simulink model "manual_waveInput"  (R2023a)
settings: Solver=FixedStepAuto  StartTime=0.0  StopTime=inf  FixedStep=0.01  RelTol=1e-3  EnableMultiTasking=on
undefined symbols (not defined in the file): dev, Main, mf, P0, pwm_output0, Q, R, Rbody_frd, Ts_EKF_integr, Ts_EKF_meas, Ts_slk, x0EKF
libraries: simulink_extras x6, px4Sensorslib x4, sharedtransform x4, px4lib x1, px4uORBlib x1
settings Model: SimulationMode=external  ExtModeTrigDuration=10  Creator=ArriGE66  LastModifiedBy=User
settings SolverCC: PositivePriorityOrder=on
settings OptimizationCC: EnhancedBackFolding=on  PassReuseOutputArgsAs=Individual arguments  ZeroExternalMemoryAtStartup=off  ZeroInternalMemoryAtStartup=off  MaxStackSize=64  OptimizeBlockOrder=speed  DifferentSizesBufferReuse=on  OptimizationCustomize=off  EfficientTunableParamExpr=on
settings DebuggingCC: ParameterTunabilityLossMsg=error
settings HardwareCC: ProdBitPerPointer=32  ProdBitPerSizeT=32  ProdBitPerPtrDiffT=32  ProdLargestAtomicInteger=Long  ProdLargestAtomicFloat=Double  ProdWordSize=32  ProdLongLongMode=on  ProdHWDeviceType=ARM Compatible->ARM Cortex
settings SFSimCC: MATLABDynamicMemAlloc=off  SimTargetLang=C++
settings RTWCC: Description=Embedded Coder  SystemTargetFile=ert.tlc  HardwareBoard=PX4 Cube Orange  TemplateMakefile=ert_default_tmf  Toolchain=GNU Tools for PX4 Autopilots  TargetLang=C++
settings CodeAppCC: ForceParamTrailComments=on  IgnoreCustomStorageClasses=off  OperatorAnnotations=on  SimulinkDataObjDesc=on  SFDataObjDesc=on  InsertBlockDesc=on
settings ERTTargetCC: ExtMode=on  ExtModeTransport=3  ExtModeStaticAlloc=on  ExtModeStaticAllocSize=1024  ExtModeMexFile=ext_xcp  ExtModeMexArgs=1 COM10 3000000  ExtModeIntrfLevel=Level2 - Open

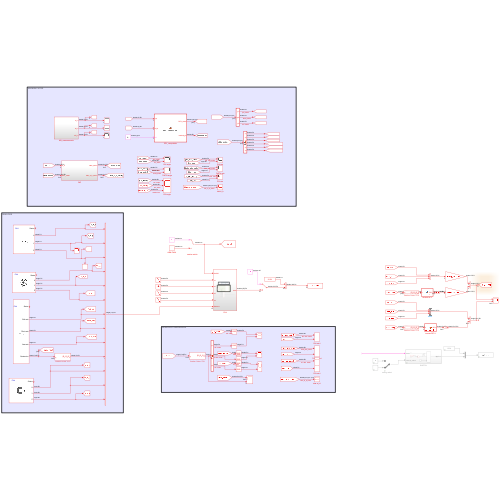
[thumbnail: Simulink's stored preview of the top-level diagram]
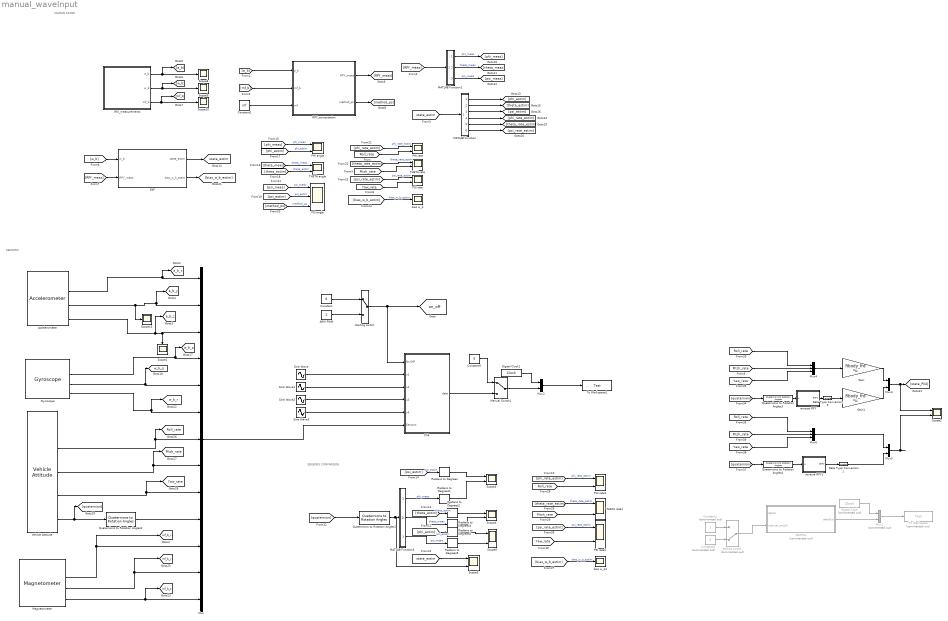
== system manual_waveInput ==
  note: KALMAN FILTER
  note: SENSORS
  note: SENSORS COMPARISON
  ARM PWM : Constant  OutDataTypeStr=boolean  SampleTime=0.01
  Accelerometer : px4Sensorslib/Accelerometer  uorbTimeStamp=off  BlockingMode=off  BlockTimeout=1e-3  sampleTime=1/100
  Constant : Constant  Value=0  OutDataTypeStr=boolean
  Constant1 : Constant  Commented=on  OutDataTypeStr=boolean
  Constant2 : Constant  Value=mf
  Constant3 : Constant  Commented=on  Value=0  OutDataTypeStr=boolean
  Constant5 : Constant  Value=0  OutDataTypeStr=boolean
  Data Type Conversion1 : DataTypeConversion  OutDataTypeStr=single  SaturateOnIntegerOverflow=off  RndMeth=Floor
  Data Type Conversion5 : DataTypeConversion  OutDataTypeStr=single  SaturateOnIntegerOverflow=off  RndMeth=Floor
  Digital Clock : DigitalClock  Commented=on  SampleTime=0.01
  Digital Clock1 : DigitalClock  SampleTime=0.01
  EKF : Subsystem
  Gain : Gain  Gain=Rbody_frd  Multiplication=Matrix(K*u) (u vector)
  Gain1 : Gain  Gain=Rbody_frd  Multiplication=Matrix(K*u) (u vector)
  Gyroscope : px4Sensorslib/Gyroscope  uorbTimeStamp=off  BlockingMode=off  BlockTimeout=1e-3  sampleTime=1/100
  IMU_measurements : Subsystem
  MATLAB Function : MATLAB Function  TreatAsAtomicUnit=on
  MATLAB Function1 : MATLAB Function  TreatAsAtomicUnit=on
  MATLAB Function3 : MATLAB Function  TreatAsAtomicUnit=on
  Magnetometer : px4Sensorslib/Magnetometer  uorbTimeStamp=off  BlockingMode=off  BlockTimeout=1e-3  sampleTime=0.01
  Manual Switch1 : ManualSwitch
  Mux : Mux  Inputs=13
  Mux1 : Mux  Commented=on  Inputs=2
  Mux2 : Mux  Inputs=2
  Mux3 : Mux  Inputs=2
  Mux4 : Mux  Inputs=3
  Mux5 : Mux  Inputs=2
  Mux6 : Mux  Inputs=3
  PHI angle : Scope  NumInputPorts=2
  PHI rate : Scope  NumInputPorts=2
  PHI rate1 : Scope  NumInputPorts=2
  PSI angle : Scope  NumInputPorts=3
  PSI rate : Scope  NumInputPorts=2
  PSI rate1 : Scope  NumInputPorts=2
  PX4 : Subsystem
  Quaternions to Rotation Angles{1..4} (4 alike) : sharedtransform/Quaternions to Rotation Angles  rotationOrder=ZYX  aMode=aMode
  RPY_computation : MATLAB Function  TreatAsAtomicUnit=on
  Radians to Degrees{,1..5} (6 alike) : simulink_extras/Transformations/Radians to Degrees
  SWITCH : Subsystem  Commented=on
  Scope{1,8..10,13} (5 alike) : Scope
  Scope{2..6} (5 alike) : Scope  NumInputPorts=2
  Sine Wave : Sin  Amplitude=0  SampleTime=0.01
  Sine Wave1 : Sin  Amplitude=0  Phase=pi/2  SampleTime=0.01
  Sine Wave2 : Sin  Amplitude=200  Bias=300  SampleTime=0.01
  Sine Wave3 : Sin  Amplitude=200  Bias=300  Phase=pi/2  SampleTime=0.01
  THETA angle : Scope  NumInputPorts=2
  THETA rate : Scope  NumInputPorts=2
  THETA rate1 : Scope  NumInputPorts=2
  To Workspace : ToWorkspace  Commented=on  VariableName=Test  SampleTime=0.01
      settings: Save2DSignal=2-D array (concatenate along first dimension)
  To Workspace1 : ToWorkspace  VariableName=Test  SampleTime=-1
      settings: Save2DSignal=2-D array (concatenate along first dimension)
  Vehicle Attitude : px4Sensorslib/Vehicle Attitude  rollRate=on  pitchRate=on  yawRate=on  quaternion=on  uorbTimeStamp=off  BlockingMode=off  BlockTimeout=0.001  sampleTime=1/100
  bias w_b : Scope
  bias w_b1 : Scope
  ending switch : ManualSwitch  Commented=on  CurrentSetting=0
  reverse RPY : MATLAB Function  TreatAsAtomicUnit=on
  reverse RPY1 : MATLAB Function  TreatAsAtomicUnit=on
  starting switch : ManualSwitch
  tag scope: Pitch_rate=global, Roll_rate=global, Yaw_rate=global, a_b_x=global, a_b_y=global, a_b_z=global, mf_b_x=global, mf_b_y=global, mf_b_z=global, on_off=global, state_estim=global, w_b_p=global, w_b_q=global, w_b_r=global
  wires:
  Vehicle Attitude/3 -> [Pitch_rate], Mux/8
  Vehicle Attitude/2 -> [Roll_rate], Mux/7
  ARM PWM/1 -> starting switch/2
  Constant/1 -> starting switch/1
  Gyroscope/4 -> [w_b_r], Mux/6
  Gyroscope/3 -> [w_b_q], Mux/5
  Gyroscope/2 -> [w_b_p], Mux/4
  Accelerometer/2 -> [a_b_x], Mux/1
  Accelerometer/3 -> Scope13/1, [a_b_y], Mux/2
  Accelerometer/4 -> [a_b_z], Mux/3, Scope1/1
  Vehicle Attitude/4 -> [Yaw_rate], Mux/9
  Magnetometer/2 -> [mf_b_x], Mux/11
  Magnetometer/3 -> Mux/12, [mf_b_y]
  Magnetometer/4 -> [mf_b_z], Mux/13
  MATLAB Function1/2(y2) -> [theta_meas]  "theta_meas"
  [bias_w_b_estim] -> bias w_b/1  "bias_w_b_estim"
  [mf_b] -> RPY_computation/2(mf_b)
  [theta_estim] -> THETA angle/2  "theta_estim"
  MATLAB Function1/1(y1) -> [phi_meas]  "phi_meas"
  [RPY_meas] -> EKF/2(RPY_meas)
  [psi_meas] -> PSI angle/1  "psi_meas"
  [method_ps] -> PSI angle/3  "method_ps"
  IMU_measurements/2(w_b) -> Scope9/1, [w_b]
  [psi_estim] -> PSI angle/2  "psi_estim"
  MATLAB Function1/3(y3) -> [psi_meas]  "psi_meas"
  [RPY_meas] -> MATLAB Function1/1(u)
  [theta_meas] -> THETA angle/1  "theta_meas"
  [phi_rate_estim] -> PHI rate/1  "phi_rate_estim"
  [psi_rate_estim] -> PSI rate/1  "psi_rate_estim"
  [theta_rate_estim] -> THETA rate/1  "theta_rate_estim"
  EKF/1(state_estim) -> [state_estim]
  [phi_estim] -> PHI angle/2  "phi_estim"
  [w_b] -> EKF/1(w_b)
  IMU_measurements/3(mf_b) -> [mf_b], Scope10/1
  Constant2/1 -> RPY_computation/3(mf)
  IMU_measurements/1(a_b) -> [a_b], Scope8/1
  RPY_computation/2(method_ps) -> [method_ps]
  [a_b] -> RPY_computation/1(a_b)
  EKF/2(bias_w_b_estim) -> [bias_w_b_estim]
  [phi_meas] -> PHI angle/1  "phi_meas"
  RPY_computation/1(RPY_meas) -> [RPY_meas]
  starting switch/1 -> PX4/1(On/Off), [on_off]
  Mux/1 -> PX4/6(Sensors)
  [state_estim] -> MATLAB Function/1(u)
  MATLAB Function/1(y1) -> [phi_estim]
  MATLAB Function/2(y2) -> [theta_estim]
  MATLAB Function/3(y3) -> [psi_estim]
  MATLAB Function/4(y4) -> [phi_rate_estim]
  MATLAB Function/5(y5) -> [theta_rate_estim]
  MATLAB Function/6(y6) -> [psi_rate_estim]
  Sine Wave/1 -> PX4/2(u1)
  Sine Wave1/1 -> PX4/3(u2)
  Sine Wave2/1 -> PX4/4(u3)
  Sine Wave3/1 -> PX4/5(u4)
  [Roll_rate] -> PHI rate/2
  [Pitch_rate] -> THETA rate/2
  [Yaw_rate] -> PSI rate/2
  [bias_w_b_estim] -> bias w_b1/1  "bias_w_b_estim"
  [psi_rate_estim] -> PSI rate1/1  "psi_rate_estim"
  Radians to Degrees2/1 -> Scope4/1
  [state_estim] -> Scope6/1
  [phi_estim] -> Radians to Degrees4/1  "phi_estim"
  MATLAB Function3/3(y3) -> Radians to Degrees5/1  "psi_meas"
  MATLAB Function3/1(y1) -> Radians to Degrees1/1  "phi_meas"
  [theta_estim] -> Radians to Degrees2/1  "theta_estim"
  Radians to Degrees1/1 -> Scope3/2
  Quaternions to Rotation Angles1/1 -> Scope6/2, MATLAB Function3/1(u)
  Radians to Degrees3/1 -> Scope4/2
  Radians to Degrees5/1 -> Scope5/2
  MATLAB Function3/2(y2) -> Radians to Degrees3/1  "theta_meas"
  Radians to Degrees/1 -> Scope3/1
  Radians to Degrees4/1 -> Scope5/1
  [Roll_rate] -> PHI rate1/2
  [psi_estim] -> Radians to Degrees/1  "psi_estim"
  [Yaw_rate] -> PSI rate1/2
  [theta_rate_estim] -> THETA rate1/1  "theta_rate_estim"
  [quaternion] -> Quaternions to Rotation Angles1/1
  [Pitch_rate] -> THETA rate1/2
  [phi_rate_estim] -> PHI rate1/1  "phi_rate_estim"
  Vehicle Attitude/5 -> [quaternion], Quaternions to Rotation Angles2/1
  Quaternions to Rotation Angles2/1 -> Mux/10
  Constant3/1 -> ending switch/2
  ? -> SWITCH/1(dataIn)
  ending switch/1 -> SWITCH/2(manual_switch)
  Constant1/1 -> ending switch/1
  Mux1/1 -> To Workspace/1
  Digital Clock/1 -> Mux1/1
  SWITCH/1(dataOut) -> Mux1/2
  Mux2/1 -> To Workspace1/1
  Constant5/1 -> Manual Switch1/1
  Digital Clock1/1 -> Mux2/1
  Manual Switch1/1 -> Mux2/2
  PX4/1(data) -> Manual Switch1/2
  [Pitch_rate] -> Mux4/2
  [Yaw_rate] -> Mux4/3
  Mux3/1 -> Scope2/1, [state_PX4]
  Data Type Conversion5/1 -> Gain1/1
  [Roll_rate] -> Mux4/1
  Quaternions to Rotation Angles3/1 -> reverse RPY/1(u)
  reverse RPY/1(RPY) -> Data Type Conversion5/1
  Gain/1 -> Mux3/1
  [quaternion] -> Quaternions to Rotation Angles3/1
  Mux4/1 -> Gain/1
  Gain1/1 -> Mux3/2
  Data Type Conversion1/1 -> Mux5/2
  Mux6/1 -> Mux5/1
  reverse RPY1/1(RPY) -> Data Type Conversion1/1
  Quaternions to Rotation Angles4/1 -> reverse RPY1/1(u)
  [quaternion] -> Quaternions to Rotation Angles4/1
  [Roll_rate] -> Mux6/1
  Mux5/1 -> Scope2/2
  [Pitch_rate] -> Mux6/2
  [Yaw_rate] -> Mux6/3

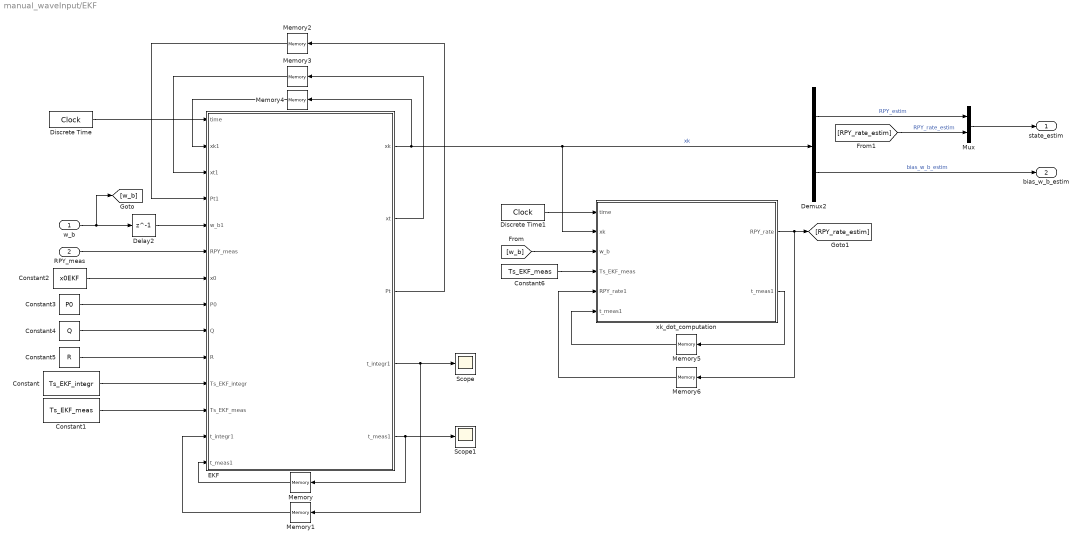
== system manual_waveInput/EKF ==
  w_b : Inport
  RPY_meas : Inport  Port=2
  Constant : Constant  Value=Ts_EKF_integr
  Constant1 : Constant  Value=Ts_EKF_meas
  Constant2 : Constant  Value=x0EKF
  Constant3 : Constant  Value=P0
  Constant4 : Constant  Value=Q
  Constant5 : Constant  Value=R
  Constant6 : Constant  Value=Ts_EKF_meas
  Delay2 : Delay  DelayLength=1  SampleTime=Ts_EKF_integr
  Demux2 : Demux  Outputs=2
  Discrete Time : DigitalClock  SampleTime=Ts_slk
  Discrete Time1 : DigitalClock  SampleTime=Ts_slk
  EKF : MATLAB Function  TreatAsAtomicUnit=on
  Memory{,1..6} (7 alike) : Memory
  Mux : Mux  Inputs=2
  Scope : Scope
  Scope1 : Scope
  xk_dot_computation : MATLAB Function  TreatAsAtomicUnit=on
  state_estim : Outport
  bias_w_b_estim : Outport  Port=2
  wires:
  w_b/1 -> Delay2/1, [w_b]
  Constant4/1 -> EKF/9(Q)
  Constant2/1 -> EKF/7(x0)
  Constant5/1 -> EKF/10(R)
  Memory/1 -> EKF/14("t_meas1 ")
  EKF/2(xt) -> Memory3/1
  Memory2/1 -> EKF/4(Pt1)
  EKF/3(Pt) -> Memory2/1
  RPY_meas/1 -> EKF/6(RPY_meas)
  Discrete Time/1 -> EKF/1(time)
  Memory3/1 -> EKF/3(xt1)
  Memory1/1 -> EKF/13("t_integr1 ")
  Constant3/1 -> EKF/8(P0)
  EKF/5(t_meas1) -> Scope1/1, Memory/1
  EKF/4(t_integr1) -> Scope/1, Memory1/1
  Delay2/1 -> EKF/5(w_b1)
  Constant/1 -> EKF/11(Ts_EKF_integr)
  Constant1/1 -> EKF/12(Ts_EKF_meas)
  Memory4/1 -> EKF/2(xk1)
  xk_dot_computation/2(t_meas1) -> Memory5/1
  Memory5/1 -> xk_dot_computation/6("t_meas1 ")
  Memory6/1 -> xk_dot_computation/5(RPY_rate1)
  xk_dot_computation/1(RPY_rate) -> [RPY_rate_estim], Memory6/1
  [w_b] -> xk_dot_computation/3(w_b)
  Discrete Time1/1 -> xk_dot_computation/1(time)
  Demux2/2 -> bias_w_b_estim/1  "bias_w_b_estim"
  Demux2/1 -> Mux/1  "RPY_estim"
  EKF/1(xk) -> xk_dot_computation/2(xk), Demux2/1, Memory4/1  "xk"
  [RPY_rate_estim] -> Mux/2  "RPY_rate_estim"
  Constant6/1 -> xk_dot_computation/4(Ts_EKF_meas)
  Mux/1 -> state_estim/1

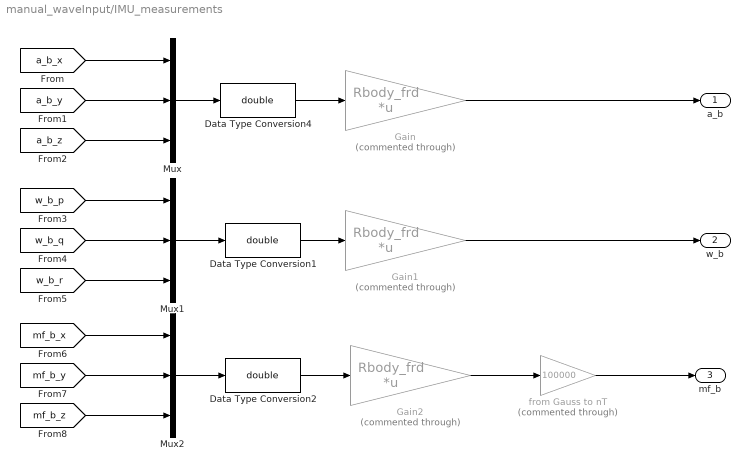
== system manual_waveInput/IMU_measurements ==
  Data Type Conversion1 : DataTypeConversion  OutDataTypeStr=double  SaturateOnIntegerOverflow=off  RndMeth=Floor
  Data Type Conversion2 : DataTypeConversion  OutDataTypeStr=double  SaturateOnIntegerOverflow=off  RndMeth=Floor
  Data Type Conversion4 : DataTypeConversion  OutDataTypeStr=double  SaturateOnIntegerOverflow=off  RndMeth=Floor
  Gain : Gain  Commented=through  Gain=Rbody_frd  Multiplication=Matrix(K*u) (u vector)
  Gain1 : Gain  Commented=through  Gain=Rbody_frd  Multiplication=Matrix(K*u) (u vector)
  Gain2 : Gain  Commented=through  Gain=Rbody_frd  Multiplication=Matrix(K*u) (u vector)
  Mux : Mux  Inputs=3
  Mux1 : Mux  Inputs=3
  Mux2 : Mux  Inputs=3
  from Gauss to nT : Gain  Commented=through  Gain=100000
  a_b : Outport
  w_b : Outport  Port=2
  mf_b : Outport  Port=3
  wires:
  Gain2/1 -> from Gauss to nT/1
  Mux2/1 -> Data Type Conversion2/1
  [a_b_x] -> Mux/1
  [a_b_y] -> Mux/2
  [a_b_z] -> Mux/3
  Mux/1 -> Data Type Conversion4/1
  Mux1/1 -> Data Type Conversion1/1
  [w_b_p] -> Mux1/1
  [w_b_r] -> Mux1/3
  [w_b_q] -> Mux1/2
  [mf_b_x] -> Mux2/1
  [mf_b_z] -> Mux2/3
  [mf_b_y] -> Mux2/2
  Gain/1 -> a_b/1
  Gain1/1 -> w_b/1
  from Gauss to nT/1 -> mf_b/1
  Data Type Conversion4/1 -> Gain/1
  Data Type Conversion1/1 -> Gain1/1
  Data Type Conversion2/1 -> Gain2/1

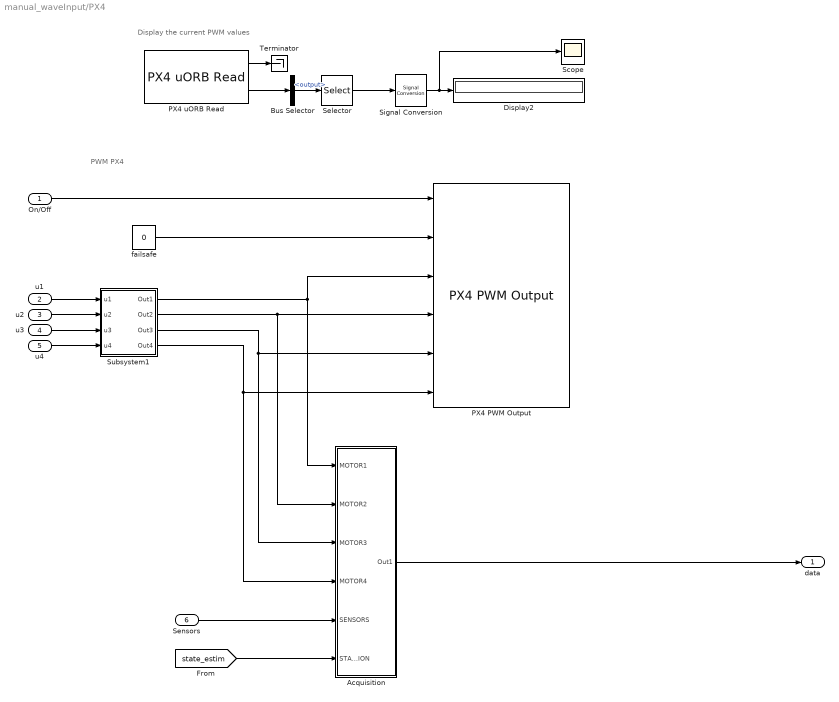
== system manual_waveInput/PX4 ==
  note: PWM PX4
  note: Display the current PWM values
  On/Off : Inport
  u1 : Inport  Port=2
  u2 : Inport  Port=3
  u3 : Inport  Port=4
  u4 : Inport  Port=5
  Sensors : Inport  Port=6
  Acquisition : Subsystem
  Bus Selector : BusSelector  OutputSignals=output
  Display2 : Display
  PX4 PWM Output : px4lib/PX4 PWM Output  pwmDevice=Main (/dev/pwm_output0)  pwmChannel1_=on  pwmChannel2_=on  pwmChannel3_=on  pwmChannel4_=on  pwmChannel5_=off  pwmChannel6_=off  pwmChannel7_=off  pwmChannel8_=off  forceTerminateFailsafe=off  outputErrorStatus=on
  PX4 uORB Read : px4uORBlib/PX4 uORB Read  uORBTopic=actuator_outputs  selectInstance=actuator_outputs  SampleTime=0.01  BlockingMode=off  BlockTimeout=1e-3
  Scope : Scope
  Selector : Selector  InputPortWidth=16  IndexOptions=Index vector (dialog)  Indices=[1 2]  OutputSizes=1
  Signal Conversion : SignalConversion  OverrideOpt=off
  Subsystem1 : Subsystem
  Terminator : Terminator
  failsafe : Constant  Value=0  OutDataTypeStr=boolean  SampleTime=0.01
  data : Outport
  wires:
  failsafe/1 -> PX4 PWM Output/2
  Subsystem1/2(Out2) -> Acquisition/2(MOTOR2), PX4 PWM Output/4
  Subsystem1/4(Out4) -> Acquisition/4(MOTOR4), PX4 PWM Output/6
  Subsystem1/3(Out3) -> Acquisition/3(MOTOR3), PX4 PWM Output/5
  Subsystem1/1(Out1) -> Acquisition/1(MOTOR1), PX4 PWM Output/3
  Sensors/1 -> Acquisition/5(SENSORS)
  On/Off/1 -> PX4 PWM Output/1
  u4/1 -> Subsystem1/4(u4)
  Acquisition/1(Out1) -> data/1
  u1/1 -> Subsystem1/1(u1)
  u2/1 -> Subsystem1/2(u2)
  u3/1 -> Subsystem1/3(u3)
  [state_estim] -> Acquisition/6(STATE ESTIMATION)
  Selector/1 -> Signal Conversion/1
  PX4 uORB Read/2 -> Bus Selector/1
  Signal Conversion/1 -> Scope/1, Display2/1
  Bus Selector/1 -> Selector/1  "<output>"
  PX4 uORB Read/1 -> Terminator/1

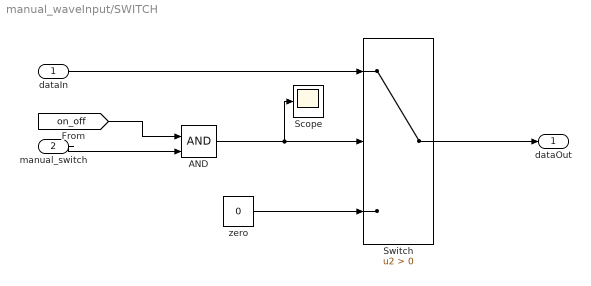
== system manual_waveInput/SWITCH ==
  dataIn : Inport
  manual_switch : Inport  Port=2
  AND : Logic  IconShape=distinctive  AllPortsSameDT=off  OutDataTypeStr=boolean
  Scope : Scope
  Switch : Switch  Criteria=u2 > Threshold  SaturateOnIntegerOverflow=off  InputSameDT=off
  zero : Constant  Value=0  OutDataTypeStr=boolean
  dataOut : Outport
  wires:
  [on_off] -> AND/1
  dataIn/1 -> Switch/1
  zero/1 -> Switch/3
  Switch/1 -> dataOut/1
  manual_switch/1 -> AND/2
  AND/1 -> Scope/1, Switch/2

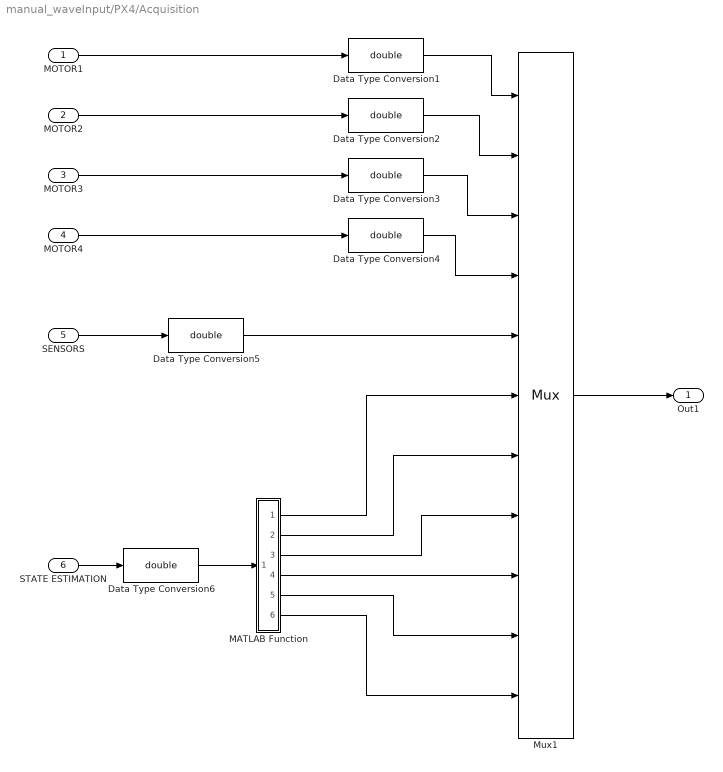
== system manual_waveInput/PX4/Acquisition ==
  MOTOR1 : Inport
  MOTOR2 : Inport  Port=2
  MOTOR3 : Inport  Port=3
  MOTOR4 : Inport  Port=4
  SENSORS : Inport  Port=5
  STATE ESTIMATION : Inport  Port=6
  Data Type Conversion{1..6} (6 alike) : DataTypeConversion  OutDataTypeStr=double  SaturateOnIntegerOverflow=off  RndMeth=Floor
  MATLAB Function : MATLAB Function  TreatAsAtomicUnit=on
  Mux1 : Mux  Inputs=11
      settings: DisplayOption=signals
  Out1 : Outport
  wires:
  MOTOR2/1 -> Data Type Conversion2/1
  Data Type Conversion1/1 -> Mux1/1
  Data Type Conversion3/1 -> Mux1/3
  Data Type Conversion4/1 -> Mux1/4
  Data Type Conversion2/1 -> Mux1/2
  MOTOR3/1 -> Data Type Conversion3/1
  STATE ESTIMATION/1 -> Data Type Conversion6/1
  Mux1/1 -> Out1/1
  SENSORS/1 -> Data Type Conversion5/1
  MOTOR1/1 -> Data Type Conversion1/1
  MOTOR4/1 -> Data Type Conversion4/1
  MATLAB Function/1(y1) -> Mux1/6
  MATLAB Function/6(y6) -> Mux1/11
  MATLAB Function/5(y5) -> Mux1/10
  MATLAB Function/4(y4) -> Mux1/9
  MATLAB Function/2(y2) -> Mux1/7
  Data Type Conversion6/1 -> MATLAB Function/1(u)
  MATLAB Function/3(y3) -> Mux1/8
  Data Type Conversion5/1 -> Mux1/5

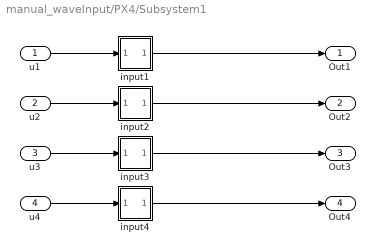
== system manual_waveInput/PX4/Subsystem1 ==
  u1 : Inport
  u2 : Inport  Port=2
  u3 : Inport  Port=3
  u4 : Inport  Port=4
  input1 : Subsystem
  input2 : Subsystem
  input3 : Subsystem
  input4 : Subsystem
  Out1 : Outport
  Out2 : Outport  Port=2
  Out3 : Outport  Port=3
  Out4 : Outport  Port=4
  wires:
  u2/1 -> input2/1(In1)
  u1/1 -> input1/1(In1)
  input1/1(Out1) -> Out1/1
  u4/1 -> input4/1(In1)
  input4/1(Out1) -> Out4/1
  input2/1(Out1) -> Out2/1
  u3/1 -> input3/1(In1)
  input3/1(Out1) -> Out3/1

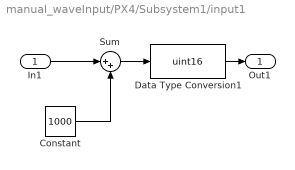
== system manual_waveInput/PX4/Subsystem1/input1 ==
  In1 : Inport
  Constant : Constant  Value=1000  SampleTime=0.01
  Data Type Conversion1 : DataTypeConversion  OutDataTypeStr=uint16  SaturateOnIntegerOverflow=off  RndMeth=Floor
  Sum : Sum  Inputs=|++
  Out1 : Outport
  wires:
  Sum/1 -> Data Type Conversion1/1
  In1/1 -> Sum/1
  Constant/1 -> Sum/2
  Data Type Conversion1/1 -> Out1/1

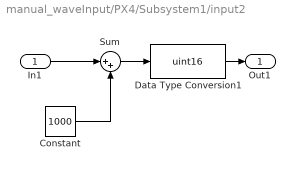
== system manual_waveInput/PX4/Subsystem1/input2 ==
  In1 : Inport
  Constant : Constant  Value=1000  SampleTime=0.01
  Data Type Conversion1 : DataTypeConversion  OutDataTypeStr=uint16  SaturateOnIntegerOverflow=off  RndMeth=Floor
  Sum : Sum  Inputs=|++
  Out1 : Outport
  wires:
  Sum/1 -> Data Type Conversion1/1
  In1/1 -> Sum/1
  Constant/1 -> Sum/2
  Data Type Conversion1/1 -> Out1/1

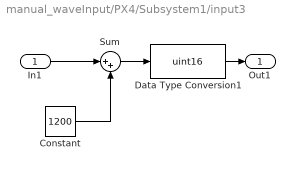
== system manual_waveInput/PX4/Subsystem1/input3 ==
  In1 : Inport
  Constant : Constant  Value=1200  SampleTime=0.01
  Data Type Conversion1 : DataTypeConversion  OutDataTypeStr=uint16  SaturateOnIntegerOverflow=off  RndMeth=Floor
  Sum : Sum  Inputs=|++
  Out1 : Outport
  wires:
  Sum/1 -> Data Type Conversion1/1
  In1/1 -> Sum/1
  Constant/1 -> Sum/2
  Data Type Conversion1/1 -> Out1/1

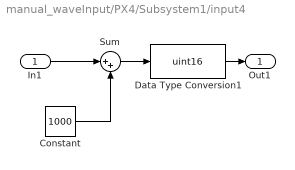
== system manual_waveInput/PX4/Subsystem1/input4 ==
  In1 : Inport
  Constant : Constant  Value=1000  SampleTime=0.01
  Data Type Conversion1 : DataTypeConversion  OutDataTypeStr=uint16  SaturateOnIntegerOverflow=off  RndMeth=Floor
  Sum : Sum  Inputs=|++
  Out1 : Outport
  wires:
  Sum/1 -> Data Type Conversion1/1
  In1/1 -> Sum/1
  Constant/1 -> Sum/2
  Data Type Conversion1/1 -> Out1/1

== matlab function manual_waveInput/reverse RPY1 ==
  data: u input; RPY output
function RPY = reverse_RPY(u)
RPY = zeros(3,1);
RPY(1) = u(3);
RPY(2) = u(2);
RPY(3) = u(1);

== matlab function manual_waveInput/MATLAB Function3 ==
  data: u input; y1 output; y2 output; y3 output
function [y1,y2,y3] = fcn(u)

y1 = u(1);
y2 = u(2);
y3 = u(3);

== matlab function manual_waveInput/reverse RPY ==
  data: u input; RPY output
function RPY = reverse_RPY(u)
RPY = zeros(3,1);
RPY(1) = u(3);
RPY(2) = u(2);
RPY(3) = u(1);

== matlab function manual_waveInput/MATLAB Function1 ==
  data: u input; y1 output; y2 output; y3 output
function [y1,y2,y3] = fcn(u)

y1 = u(1);
y2 = u(2);
y3 = u(3);

== matlab function manual_waveInput/MATLAB Function ==
  data: u input; y1 output; y2 output; y3 output; y4 output; y5 output; y6 output
function [y1,y2,y3,y4,y5,y6] = fcn(u)

y1 = u(1);
y2 = u(2);
y3 = u(3);
y4 = u(4);
y5 = u(5);
y6 = u(6);

== matlab function manual_waveInput/PX4/Acquisition/MATLAB Function ==
  data: u input; y1 output; y2 output; y3 output; y4 output; y5 output; y6 output
function [y1,y2,y3,y4,y5,y6] = fcn(u)

y1 = u(1);
y2 = u(2);
y3 = u(3);
y4 = u(4);
y5 = u(5);
y6 = u(6);

== matlab function manual_waveInput/RPY_computation ==
  data: a_b input; mf_b input; RPY_meas output; mf input; method_ps output
function [RPY_meas,method_ps]   = RPY_computation(a_b,mf_b,mf)
% description:
% - a_b             = measured linear acceleration in body-frame
% - w_b             = measured angular velocity in body-frame
% - mf_b            = measured magnetic field in body-frame
% - mf              = measured magnetic field in body-inertia
% - a_b_disturbe    = linear velocity measurement-noise
% - w_b_disturbe    = angular velocity measurement-noise
% - mf_b_disturbe   = magnetic field measurement-noise

% -------------------------------------------------------------------------------------------
% observation: the following computation works only if the angles
% phi,theta,psy are withing angles (-pi/2,+pi/2) (this is an open set, pi/2 is excluded)
% -------------------------------------------------------------------------------------------

a_b = -1*a_b;       % need to adjust the sign to use atan2() function correctly
mf_u = mf(3,1);     % magnetic field in up direction (z-dir in inertia frame)

% phi computation
ph_meas = atan2(a_b(2), a_b(3));
sph = sin(ph_meas);
cph = cos(ph_meas);

% theta computation
th_meas = atan2(-a_b(1), (a_b(2)*sph + a_b(3)*cph));
sth = sin(th_meas);
cth = cos(th_meas);

% psi computation
if abs(sin(th_meas)) > 0.1  % sin(th) != 0 
    method_ps = 1;
    ps_meas_numerator   = (sth*cph*mf_b(2) - sth*sph*mf_b(3))/(-sth);       % don't modify
    ps_meas_denominator = (-sph*mf_b(2) - cph*mf_b(3) + cth*mf_u)/(-sth);   % don't modify
    ps_meas = atan2(ps_meas_numerator, ps_meas_denominator);
else                        % sin(th) == 0
    method_ps = 2;
    ps_meas_numerator   = (mf_b(2) - cth*sph*mf_u)*(-cth);
    ps_meas_denominator = cph*mf_b(1);
    ps_meas = atan2(ps_meas_numerator, ps_meas_denominator);
end
RPY_meas = [ph_meas;th_meas;ps_meas];

== matlab function manual_waveInput/EKF/EKF ==
  data: time input; xk1 input; xt1 input; Pt1 input; w_b1 input; RPY_meas input; x0 input; P0 input; Q input; R input; Ts_EKF_integr input; Ts_EKF_meas input; xk output; t_integr1 input; t_meas1 input; xt output; Pt output; t_integr1 output; t_meas1 output
function [xk,xt,Pt,t_integr1,t_meas1] = EKF(time,xk1,xt1,Pt1,w_b1,RPY_meas,x0,P0,Q,R,Ts_EKF_integr,Ts_EKF_meas,t_integr1,t_meas1)

if time == 0
    xk = x0;
    xt = x0;
    Pt = P0;
    t_integr1 = 0;
    t_meas1 = 0;
elseif time - t_integr1 >= Ts_EKF_integr
    wp          =       w_b1(1,1);        % p-dir of angular velocity w
    wq          =       w_b1(2,1);        % q-dir of angular velocity w
    wr          =       w_b1(3,1);        % r-dir of angular velocity w

    phi         =       xt1(1,1);         %  roll angle (rad)
    theta       =       xt1(2,1);         %  pitch angle (rad)
    psi         =       xt1(3,1);         %  yaw angle (rad)  
    bias_wp     =       xt1(4,1);         % bias of p-dir of angular velocity w
    bias_wq     =       xt1(5,1);         % bias of q-dir of angular velocity w
    bias_wr     =       xt1(6,1);         % bias of r-dir of angular velocity w

    cph         =       cos(phi);
    cth         =       cos(theta);
    cps         =       cos(psi);
    sph         =       sin(phi);
    sth         =       sin(theta);
    sps         =       sin(psi);
    tth         =       sth/cth;

    % integration step
    t_integr1 = time;
    Mf = [1,    sph*tth,    cph*tth,    0,  0,  0;
          0,    cph,        -sph,       0,  0,  0;
          0,    sph/cth,    cph/cth,    0,  0,  0;
          0,    0,          0,          1,  0,  0;
          0,    0,          0,          0,  1,  0;
          0,    0,          0,          0,  0,  1;];
    Z1 = [wp-bias_wp; wq-bias_wq; wr-bias_wr; bias_wp; bias_wq; bias_wr;];
    f = Mf*Z1;
    xt = xt1 + Ts_EKF_integr*f;

    A1 = [cph*tth*(wq-bias_wq)-sph*tth*(wr-bias_wr),(sph*(wq-bias_wq)+cph*(wr-bias_wr))/cth^2,  0,  -1, -sph*tth,   -cph*tth;];
    A2 = [-sph*(wq-bias_wq)-cph*(wr-bias_wr),   0,  0,  0,  -cph,   sph;];
    A3 = [cph*(wq-bias_wq)/cth-sph*(wr-bias_wr)/cth, (sth/cth^2)*(sph*(wq-bias_wq)+cph*(wr-bias_wr)),   0,  0,  -sph/cth,   -cph/cth;];
    A4 = [0,    0,  0,  1,  0,  0;];
    A5 = [0,    0,  0,  0,  1,  0;];
    A6 = [0,    0,  0,  0,  0,  1;];
    At1 = [A1; A2; A3; A4; A5; A6;];
    Pt = Pt1 + Ts_EKF_integr*(At1*Pt1 + Pt1*At1' + Q);

    % measurement step
    if time - t_meas1 >= Ts_EKF_meas
        t_meas1 = time;
        Ck = [eye(3),zeros(3,3)];
        Lk = Pt*Ck'/(Ck*Pt*Ck' + R);
        xk = xt + Lk*(RPY_meas - Ck*xt);
        Pk = (eye(6) - Lk*Ck)*Pt;

        xt = xk;    % becomes the new xt1
        Pt = Pk;    % becomes the new Pt1
    else
        xk = xk1;    % xk1
    end
else
    xk = xt1;
    xt = xt1;
    Pt = Pt1;
end
end

== matlab function manual_waveInput/EKF/xk_dot_computation ==
  data: time input; xk input; w_b input; Ts_EKF_meas input; RPY_rate1 input; RPY_rate output; t_meas1 input; t_meas1 output
function [RPY_rate,t_meas1] = xk_dot_computation(time,xk,w_b,Ts_EKF_meas,RPY_rate1,t_meas1)
RPY_rate = zeros(3,1);
if time == 0
    t_meas1 = 0;
end
if time - t_meas1 >= Ts_EKF_meas || time == 0
    wp          =       w_b(1,1);        % p-dir of angular velocity w
    wq          =       w_b(2,1);        % q-dir of angular velocity w
    wr          =       w_b(3,1);        % r-dir of angular velocity w

    phi         =       xk(1,1);         %  roll angle (rad)
    theta       =       xk(2,1);         %  pitch angle (rad)
    psi         =       xk(3,1);         %  yaw angle (rad)  
    bias_wp     =       xk(4,1)*0;         % bias of p-dir of angular velocity w
    bias_wq     =       xk(5,1)*0;         % bias of q-dir of angular velocity w
    bias_wr     =       xk(6,1)*0;         % bias of r-dir of angular velocity w

    cph         =       cos(phi);
    cth         =       cos(theta);
    cps         =       cos(psi);
    sph         =       sin(phi);
    sth         =       sin(theta);
    sps         =       sin(psi);
    tth         =       sth/cth;

    % integration step
    t_meas1 = time;
    W_eta = [1,    sph*tth,    cph*tth;
             0,    cph,        -sph;
             0,    sph/cth,    cph/cth;];
    w_b_corrected = [wp-bias_wp; wq-bias_wq; wr-bias_wr;];
    RPY_rate = W_eta*w_b_corrected;
else
    RPY_rate = RPY_rate1;
end
end
